simulink model "solver_simulink"  (R2016b)
settings: Solver=VariableStepAuto  StartTime=0.0  StopTime=120  FixedStep=0.01  MaxStep=0.01  RelTol=1e-6  AbsTol=1e-9
undefined symbols (not defined in the file): aerodata, CM, CP, mass, rINT, T, t_step, uINT, wind
settings Model: Creator=ME-123-10  LastModifiedBy=ME-123-10

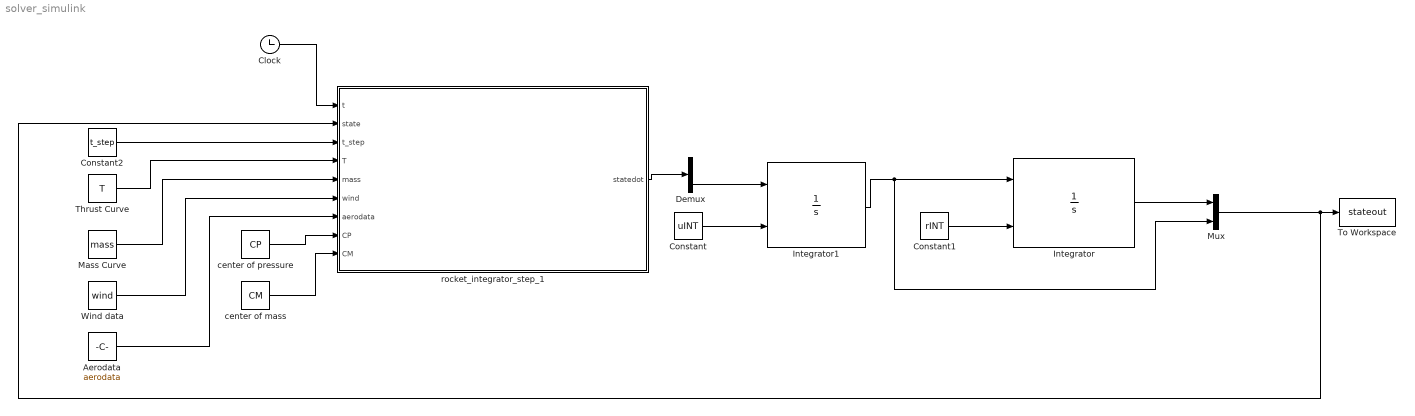
== system solver_simulink ==
  "Aerodata " : Constant  Value=aerodata
  Clock : Clock
  Constant : Constant  Value=uINT
  Constant1 : Constant  Value=rINT
  Constant2 : Constant  Value=t_step
  Demux : Demux  Outputs=2
  Integrator : Integrator  InitialConditionSource=external
  Integrator1 : Integrator  InitialConditionSource=external
  Mass Curve : Constant  Value=mass
  Mux : Mux  Inputs=2
  "Thrust Curve " : Constant  Value=T
  To Workspace : ToWorkspace  VariableName=stateout  SampleTime=-1
  Wind data : Constant  Value=wind
  "center of mass " : Constant  Value=CM
  "center of pressure " : Constant  Value=CP
  "rocket_integrator_step_1 " : MATLAB Function  TreatAsAtomicUnit=on
  wires:
  Integrator1/1 -> Mux/2, Integrator/1
  Constant/1 -> Integrator1/2
  Constant1/1 -> Integrator/2
  Clock/1 -> "rocket_integrator_step_1 "/1(t)
  "rocket_integrator_step_1 "/1(statedot) -> Demux/1
  Demux/2 -> Integrator1/1
  Mux/1 -> "rocket_integrator_step_1 "/2(state), To Workspace/1
  Integrator/1 -> Mux/1
  "Thrust Curve "/1 -> "rocket_integrator_step_1 "/4(T)
  Mass Curve/1 -> "rocket_integrator_step_1 "/5(mass)
  Constant2/1 -> "rocket_integrator_step_1 "/3(t_step)
  "Aerodata "/1 -> "rocket_integrator_step_1 "/7(aerodata)
  Wind data/1 -> "rocket_integrator_step_1 "/6(wind)
  "center of pressure "/1 -> "rocket_integrator_step_1 "/8(CP)
  "center of mass "/1 -> "rocket_integrator_step_1 "/9(CM)

== matlab function solver_simulink/rocket_integrator_step_1  ==
  data: t input; statedot output; state input; t_step input; T input; mass input; wind input; aerodata input; CP input; CM input
function statedot = dot(t, state, t_step, T, mass, wind, aerodata, CP, CM)

% avoid loading too many things. happens once each round of iterations
workspace = load('import2simulink.mat');
rocket = workspace.rocket;

% if rocket is at apogee, set theta = -180deg

statedot = zeros(6,1);      % initializes an empty vector
statedot(1:3) = state(4:6); % vx, vy, omega

% lookup current mass and calculate moment of inertia
if t <= mass(end, 1)
    k = 1; tol = t_step;
    while(1)
        delta = abs(mass(k,1)-t);
        if delta < tol; break; end
        k = k+1;
    end
    current_mass = mass(k,2);
else
    current_mass = mass(end,2);
end

I = 0.5*current_mass*rocket.OD.^2/4; % hand waves intensely

% find force/acceleration; r = state(1:3); u = state(4:6)
[f_x, f_y, moment] = forces(t, t_step, state(1:3), state(4:6), T,...
    current_mass, wind, aerodata, rocket, CP, CM);

% find acceleration
a_x = f_x/current_mass;
a_y = f_y/current_mass;
alpha = moment/I;
statedot(4) = a_x;
statedot(5) = a_y;
statedot(6) = alpha;

end
